simulink model "microreseau_irak_sous_systemes"  (R2026a)
settings: Solver=FixedStepDiscrete  StopTime=Tstop  FixedStep=Ts_model
undefined symbols (not defined in the file): Ts_model

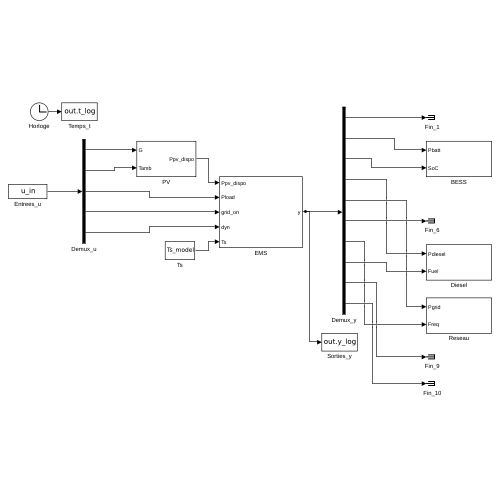
[thumbnail: Simulink's stored preview of the top-level diagram]
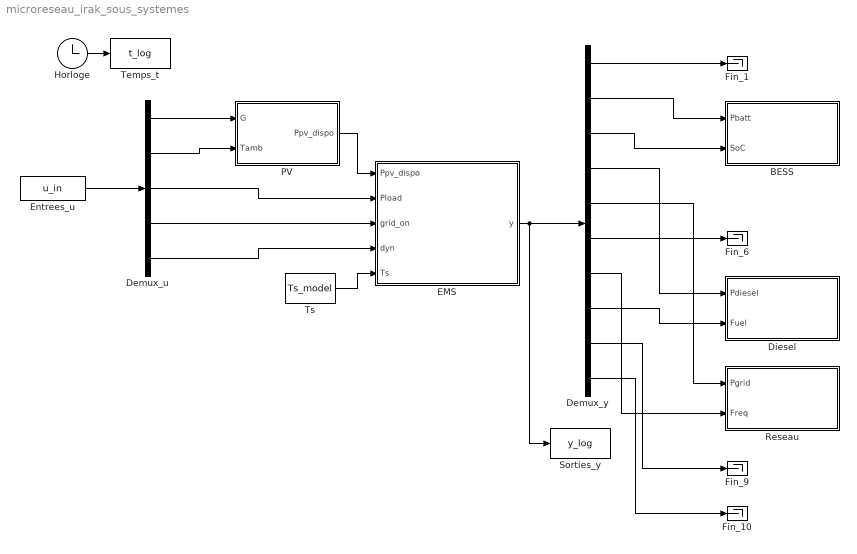
== system microreseau_irak_sous_systemes ==
  BESS : Subsystem
  Demux_u : Demux  Outputs=5
  Demux_y : Demux  Outputs=10
  Diesel : Subsystem
  EMS : Subsystem
  Entrees_u : FromWorkspace  VariableName=u_in  SampleTime=Ts_model  Interpolate=off  OutputAfterFinalValue=Holding final value
  Fin_{1,6,9..10} (4 alike) : Terminator
  Horloge : Clock
  PV : Subsystem
  Reseau : Subsystem
  Sorties_y : ToWorkspace  VariableName=y_log  SampleTime=-1
  Temps_t : ToWorkspace  VariableName=t_log  SampleTime=-1
  Ts : Constant  Value=Ts_model  SampleTime=Ts_model
  wires:
  Demux_y/10 -> Fin_10/1
  Demux_y/6 -> Fin_6/1
  Demux_y/5 -> Reseau/1(Pgrid)
  Demux_y/4 -> Diesel/1(Pdiesel)
  EMS/1(y) -> Demux_y/1, Sorties_y/1
  Entrees_u/1 -> Demux_u/1
  Horloge/1 -> Temps_t/1
  Demux_u/1 -> PV/1(G)
  Demux_y/7 -> Reseau/2(Freq)
  Demux_u/3 -> EMS/2(Pload)
  Demux_u/5 -> EMS/4(dyn)
  Demux_y/9 -> Fin_9/1
  Demux_u/2 -> PV/2(Tamb)
  Demux_u/4 -> EMS/3(grid_on)
  Demux_y/2 -> BESS/1(Pbatt)
  PV/1(Ppv_dispo) -> EMS/1(Ppv_dispo)
  Demux_y/3 -> BESS/2(SoC)
  Ts/1 -> EMS/5(Ts)
  Demux_y/8 -> Diesel/2(Fuel)
  Demux_y/1 -> Fin_1/1

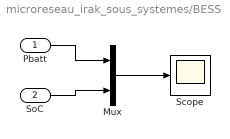
== system microreseau_irak_sous_systemes/BESS ==
  Pbatt : Inport
  SoC : Inport  Port=2
  Mux : Mux  Inputs=2
  Scope : Scope
  wires:
  Pbatt/1 -> Mux/1
  SoC/1 -> Mux/2
  Mux/1 -> Scope/1

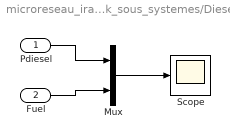
== system microreseau_irak_sous_systemes/Diesel ==
  Pdiesel : Inport
  Fuel : Inport  Port=2
  Mux : Mux  Inputs=2
  Scope : Scope
  wires:
  Pdiesel/1 -> Mux/1
  Fuel/1 -> Mux/2
  Mux/1 -> Scope/1

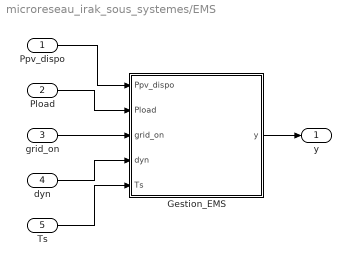
== system microreseau_irak_sous_systemes/EMS ==
  Ppv_dispo : Inport
  Pload : Inport  Port=2
  grid_on : Inport  Port=3
  dyn : Inport  Port=4
  Ts : Inport  Port=5
  Gestion_EMS : MATLAB Function  TreatAsAtomicUnit=on
  y : Outport
  wires:
  Ts/1 -> Gestion_EMS/5(Ts)
  dyn/1 -> Gestion_EMS/4(dyn)
  grid_on/1 -> Gestion_EMS/3(grid_on)
  Gestion_EMS/1(y) -> y/1
  Pload/1 -> Gestion_EMS/2(Pload)
  Ppv_dispo/1 -> Gestion_EMS/1(Ppv_dispo)

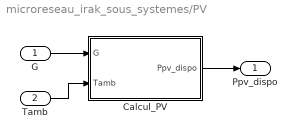
== system microreseau_irak_sous_systemes/PV ==
  G : Inport
  Tamb : Inport  Port=2
  Calcul_PV : MATLAB Function  TreatAsAtomicUnit=on
  Ppv_dispo : Outport
  wires:
  Calcul_PV/1(Ppv_dispo) -> Ppv_dispo/1
  Tamb/1 -> Calcul_PV/2(Tamb)
  G/1 -> Calcul_PV/1(G)

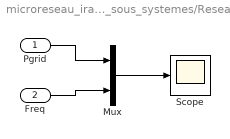
== system microreseau_irak_sous_systemes/Reseau ==
  Pgrid : Inport
  Freq : Inport  Port=2
  Mux : Mux  Inputs=2
  Scope : Scope
  wires:
  Pgrid/1 -> Mux/1
  Freq/1 -> Mux/2
  Mux/1 -> Scope/1

== matlab function microreseau_irak_sous_systemes/EMS/Gestion_EMS ==
  settings: updateMethod=DISCRETE  sampleTime=Ts_model
  data: Ppv_dispo input; y output; Pload input; grid_on input; dyn input; Ts input
function y = ems_core(Ppv_dispo, Pload, grid_on, dyn, Ts) %#codegen
% EMS_CORE  Corps du bloc "MATLAB Function" du sous-systeme EMS.
%   Conserve l'etat (SoC, frequence, carburant) entre les pas et appelle ems_step.
%   PREREQUIS : irak_params.m et ems_step.m sur le path.
%
%   y : vecteur 1x10 (voir ems_step.m)
persistent st P done
if isempty(done)
    P    = irak_params();
    st   = struct('SoC', P.BESS.SoC_init, ...
                  'freq', P.FREQ.f0, ...
                  'fuel_L', 0.0, ...
                  'f_int', 0.0);
    done = true;
end
[y, st] = ems_step(Ppv_dispo, Pload, grid_on, dyn, Ts, st, P);
end

== matlab function microreseau_irak_sous_systemes/PV/Calcul_PV ==
  settings: updateMethod=DISCRETE  sampleTime=Ts_model
  data: G input; Ppv_dispo output; Tamb input
function Ppv_dispo = pv_core(G, Tamb) %#codegen
% PV_CORE  Corps du bloc "MATLAB Function" du sous-systeme PV.
%   Charge les parametres une fois, puis appelle pv_power.
%   PREREQUIS : irak_params.m et pv_power.m sur le path.
persistent P done
if isempty(done)
    P    = irak_params();
    done = true;
end
Ppv_dispo = pv_power(G, Tamb, P);
end
